simulink model "sl_lanechange_unicycle_dynamics"  (R2013a)
settings: Solver=ode45  StartTime=0.0  StopTime=15.0  RelTol=1e-3
libraries: DiffSteer_model x2, simulink x2
settings Model: Creator=pic  LastModifiedBy=Felipe
settings DataIOCC: SignalLoggingSaveFormat=ModelDataLogs
settings OptimizationCC: ExpressionDepthLimit=2147483647
settings DebuggingCC: FcnCallInpInsideContextMsg=UseLocalSettings  StrictBusMsg=Warning
settings GRTTargetCC: CombineOutputUpdateFcns=off  GRTInterface=on

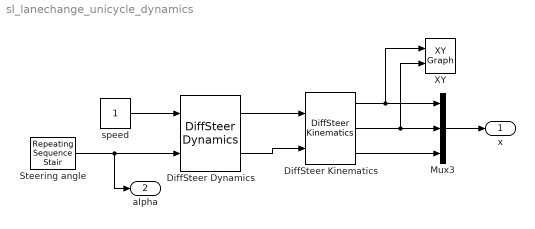
== system sl_lanechange_unicycle_dynamics ==
  DiffSteer Dynamics : DiffSteer_model/DiffSteer Dynamics  umax=0.75  wmax=1.745  dumax=0.3  dwmax=1.745  param=[0.2604 0.2509 -0.000499 0.9965 0.00263 1.0768]
  DiffSteer Kinematics : DiffSteer_model/DiffSteer Kinematics  x0=[0, 0, 0]  a=0.2  umax=0.75  wmax=1.745  dumax=0.3  dwmax=1.745
  Mux3 : Mux  Inputs=3
  Steering angle : simulink/Sources/Repeating Sequence Stair  OutValues=[0 0 0 0.5 0.5 0.5 0 0 0 -0.5 -0.5 -0.5 0 0 0 0 0]  tsamp=1  OutMin=[]  OutMax=[]  OutDataTypeStr=double  OutputDataTypeScalingMode=Specify via dialog  OutDataType=double  ConRadixGroup=Best Precision: Vector-wise  OutScaling=2^-12
  XY : simulink/Sinks/XY Graph  xmin=0  xmax=10  ymin=0  ymax=10  st=-1
  speed : Constant  VectorParams1D=off  SampleTime=0.02
  x : Outport
  alpha : Outport  Port=2
  wires:
  speed/1 -> DiffSteer Dynamics/1
  DiffSteer Kinematics/3 -> Mux3/3
  DiffSteer Kinematics/1 -> Mux3/1, XY/1
  DiffSteer Kinematics/2 -> Mux3/2, XY/2
  Mux3/1 -> x/1
  DiffSteer Dynamics/2 -> DiffSteer Kinematics/2
  DiffSteer Dynamics/1 -> DiffSteer Kinematics/1
  Steering angle/1 -> DiffSteer Dynamics/2, alpha/1
